simulink model "FM_receiver"  (Simulink 8.7)
settings: Solver=VariableStepAuto  StartTime=0.0  StopTime=0.1  RelTol=1e-3
libraries: simulink x1
settings Model: Creator=Muhammad Zubair  LastModifiedBy=Muhammad Zubair
settings DataIOCC: LimitDataPoints=off  SaveFormat=Dataset
settings DebuggingCC: UnderspecifiedInitializationDetection=Simplified  MergeDetectMultiDrivingBlocksExec=error
settings HardwareCC: ProdBitPerPointer=64  ProdLargestAtomicFloat=Float  ProdIntDivRoundTo=Zero  ProdEndianess=LittleEndian  ProdWordSize=64  ProdHWDeviceType=Intel->x86-64 (Windows64)
settings ModelReferenceCC: PropagateSignalLabelsOutOfModel=on
settings ConfigComp: CovModelRefEnable=off

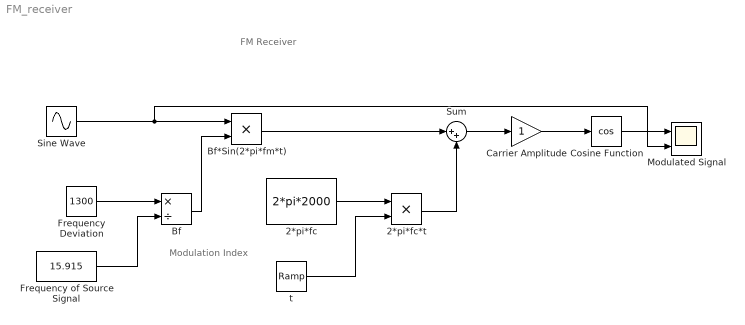
== system FM_receiver ==
  note: FM Receiver
  note: Modulation
      | Index
  2*pi*fc : Constant  Value=2*pi*2000
  2*pi*fc*t : Product  Inputs=**
  Bf : Product  Inputs=*/
  Bf*Sin(2*pi*fm*t) : Product  Inputs=**
  Carrier Amplitude : Gain
  Cosine Function : Trigonometry  Operator=cos
  Frequency Deviation : Constant  Value=1300
  Frequency of Source Signal : Constant  Value=15.915
  Modulated Signal : Scope  NumInputPorts=2
  Sine Wave : Sin  Frequency=100  SampleTime=0.0001
  Sum : Sum  Inputs=|++
  t : simulink/Sources/Ramp  slope=1  start=0  X0=0
  wires:
  Frequency Deviation/1 -> Bf/1
  Frequency of Source Signal/1 -> Bf/2
  Bf/1 -> Bf*Sin(2*pi*fm*t)/2
  Bf*Sin(2*pi*fm*t)/1 -> Sum/1
  Sum/1 -> Carrier Amplitude/1
  Carrier Amplitude/1 -> Cosine Function/1
  Cosine Function/1 -> Modulated Signal/1
  2*pi*fc/1 -> 2*pi*fc*t/1
  t/1 -> 2*pi*fc*t/2
  2*pi*fc*t/1 -> Sum/2
  Sine Wave/1 -> Modulated Signal/2, Bf*Sin(2*pi*fm*t)/1
